simulink model "sim_carroponte_OL"  (R2024b)
settings: Solver=FixedStepAuto  StartTime=0.0  StopTime=t(end)  FixedStep=mean(diff(t))  RelTol=1e-3
values from neighbouring files (symbols this model uses):
  x0 = [0 0*pi/180 0 0]'    [Progetto_Regolatore.m]    (also in carroponte_inizializzazione_solution.m)
settings Model: Creator=Giulio  LastModifiedBy=matteocorno
settings SolverCC: AlgebraicLoopSolver=TrustRegion
settings DataIOCC: ReturnWorkspaceOutputs=off
settings DebuggingCC: UnconnectedInputMsg=warning  UnconnectedOutputMsg=warning  UnconnectedLineMsg=warning  ArithmeticOperatorsInVariantConditions=warning
settings ModelReferenceCC: EnableRefExpFcnMdlSchedulingChecks=on
settings SFSimCC: SimUseLocalCustomCode=off  CustomCodeUndefinedFunction=UseInterfaceOnly
settings RTWCC: RTWUseLocalCustomCode=off  GPUComputeCapability=3.5
settings CodeAppCC: StateflowObjectComments=on

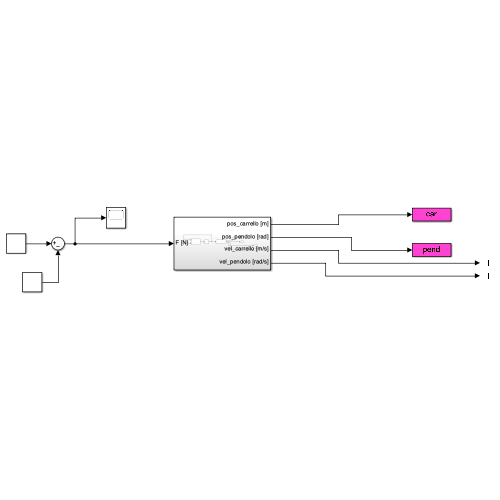
[thumbnail: Simulink's stored preview of the top-level diagram]
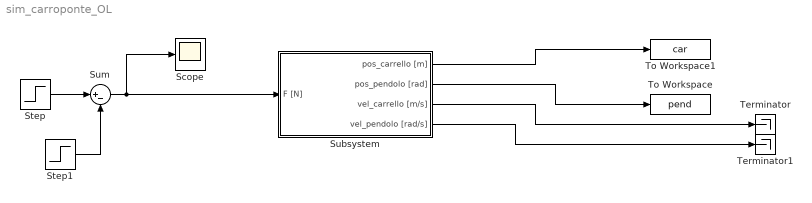
== system sim_carroponte_OL ==
  Scope : Scope
  Step : Step  After=2  SampleTime=0
  Step1 : Step  Time=2  After=2  SampleTime=0
  Subsystem : Subsystem
  Sum : Sum  Inputs=|+-
  Terminator : Terminator
  Terminator1 : Terminator
  To Workspace : ToWorkspace  VariableName=pend  SampleTime=-1
  To Workspace1 : ToWorkspace  VariableName=car  SampleTime=-1
  wires:
  Step/1 -> Sum/1
  Step1/1 -> Sum/2
  Sum/1 -> Subsystem/1(F [N]), Scope/1
  Subsystem/1(pos_carrello [m]) -> To Workspace1/1
  Subsystem/2(pos_pendolo [rad]) -> To Workspace/1
  Subsystem/3(vel_carrello [m/s]) -> Terminator/1
  Subsystem/4(vel_pendolo [rad/s]) -> Terminator1/1

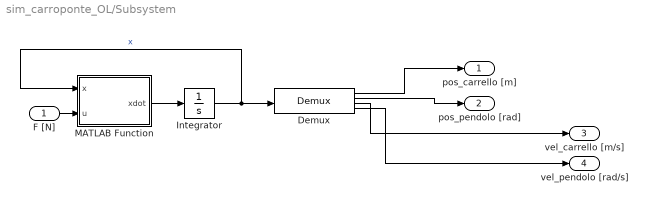
== system sim_carroponte_OL/Subsystem ==
  F [N] : Inport
  Demux : Demux
      settings: DisplayOption=none
  Integrator : Integrator  InitialCondition=x0
  MATLAB Function : MATLAB Function  TreatAsAtomicUnit=on
  pos_carrello [m] : Outport
  pos_pendolo [rad] : Outport  Port=2
  vel_carrello [m/s] : Outport  Port=3
  vel_pendolo [rad/s] : Outport  Port=4
  wires:
  Demux/1 -> pos_carrello [m]/1
  F [N]/1 -> MATLAB Function/2(u)
  Demux/3 -> vel_carrello [m/s]/1
  Demux/4 -> vel_pendolo [rad/s]/1
  Demux/2 -> pos_pendolo [rad]/1
  MATLAB Function/1(xdot) -> Integrator/1
  Integrator/1 -> MATLAB Function/1(x), Demux/1  "x"

== matlab function sim_carroponte_OL/Subsystem/MATLAB Function ==
  data: x input; u input; xdot output
function xdot = fcn(x,u)
%CARRO Summary of this function goes here
%   x = [x t xd td]

%% Parametri
l       = 0.229;
M       = 0.57;
m       = 0.119;
mtot    = M + m;

J       = 4.458e-4;
Jtot    = m*l^2 + J;

cm      = 3;            % Forza attrito massa
cp      = 1e-5;         % Forza attrito pendolo 

g = 9.81;

%% Stato
x1 = x(1);      % x
x2 = x(2);      % teta
x3 = x(3);      % x dot
x4 = x(4);      % teta dot

%% Equazioni nonlineari
xdot1 = x3;
xdot2 = x4;
xdot3 = (-Jtot*cm*x3   +   m*l*cp*cos(x2)*x4                  +   m*l*Jtot*sin(x2)*x4^2   +   m^2*l^2*g*sin(x2)*cos(x2)   +   Jtot*u)         /(Jtot*mtot - m^2*l^2*cos(x2)^2);
xdot4 = (-mtot*cp*x4   -   m^2*l^2*sin(x2)*cos(x2)*x4^2       +   cm*m*l*cos(x2)*x3       -   mtot*m*l*g*sin(x2)          -   m*l*cos(x2)*u)  /(Jtot*mtot - m^2*l^2*cos(x2)^2);

%% Uscita
xdot = [xdot1;
        xdot2;
        xdot3;
        xdot4];

end
